simulink model "Pod_Run_Simulation"  (R2020a)
settings: Solver=VariableStepAuto  StartTime=0.0  StopTime=25  RelTol=1e-3
settings Model: Creator=attir  LastModifiedBy=attir

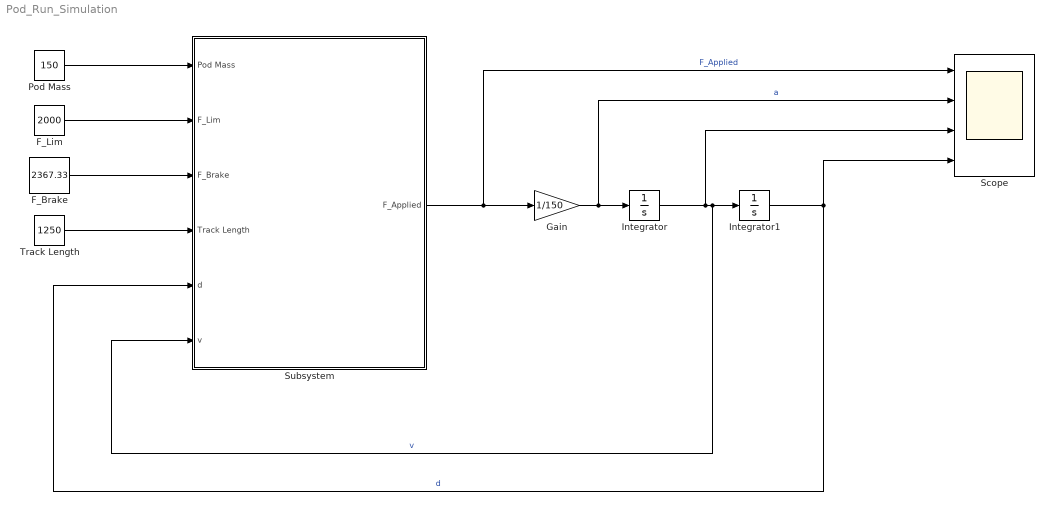
== system Pod_Run_Simulation ==
  F_Brake : Constant  Value=2367.33
  F_Lim : Constant  Value=2000
  Gain : Gain  Gain=1/150
  Integrator : Integrator
  Integrator1 : Integrator
  Pod Mass : Constant  Value=150
  Scope : Scope  NumInputPorts=4
  Subsystem : Subsystem
  Track Length : Constant  Value=1250
  wires:
  Subsystem/1(F_Applied) -> Gain/1, Scope/1  "F_Applied"
  Integrator/1 -> Scope/3, Subsystem/6(v), Integrator1/1  "v"
  Integrator1/1 -> Subsystem/5(d), Scope/4  "d"
  Gain/1 -> Scope/2, Integrator/1  "a"
  Pod Mass/1 -> Subsystem/1(Pod Mass)
  F_Lim/1 -> Subsystem/2(F_Lim)
  Track Length/1 -> Subsystem/4(Track Length)
  F_Brake/1 -> Subsystem/3(F_Brake)

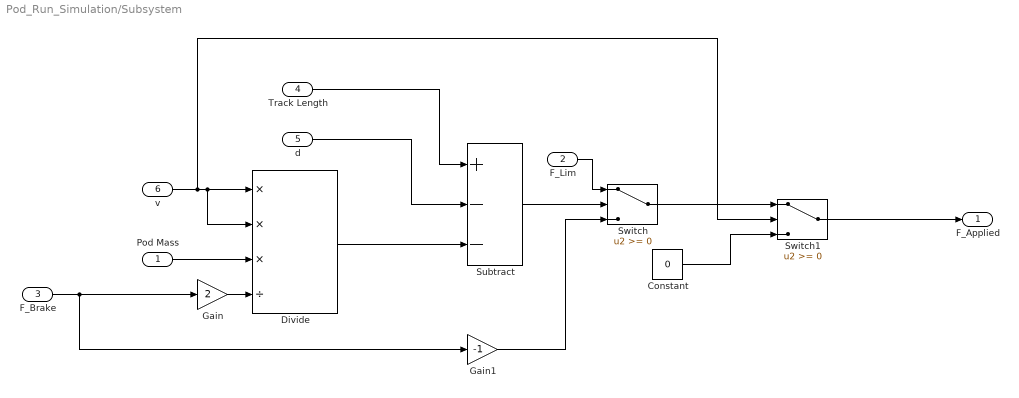
== system Pod_Run_Simulation/Subsystem ==
  Pod Mass : Inport
  F_Lim : Inport  Port=2
  F_Brake : Inport  Port=3
  Track Length : Inport  Port=4
  d : Inport  Port=5
  v : Inport  Port=6
  Constant : Constant  Value=0
  Divide : Product  Inputs=***/
  Gain : Gain  Gain=2
  Gain1 : Gain  Gain=-1
  Subtract : Sum  Inputs=+--
  Switch : Switch
  Switch1 : Switch
  F_Applied : Outport
  wires:
  v/1 -> Switch1/2, Divide/2, Divide/1
  Pod Mass/1 -> Divide/3
  Gain/1 -> Divide/4
  F_Brake/1 -> Gain/1, Gain1/1
  Track Length/1 -> Subtract/1
  d/1 -> Subtract/2
  Divide/1 -> Subtract/3
  Subtract/1 -> Switch/2
  F_Lim/1 -> Switch/1
  Gain1/1 -> Switch/3
  Switch/1 -> Switch1/1
  Switch1/1 -> F_Applied/1
  Constant/1 -> Switch1/3
